simulink model "simple_eventbased"  (R2019a)
settings: Solver=VariableStepAuto  StartTime=0.0  StopTime=10.0  RelTol=1e-3  EnableMultiTasking=on
undefined symbols (not defined in the file or in its folder): genNext, m, n
settings Model: Creator=The MathWorks, Inc.  LastModifiedBy=The MathWorks, Inc.
settings DataIOCC: LimitDataPoints=on  ReturnWorkspaceOutputs=off
settings OptimizationCC: LifeSpan=inf
settings DebuggingCC: AllowSymbolicDim=off  SFUnexpectedBacktrackingDiag=warning  SFNoUnconditionalDefaultTransitionDiag=warning  SFExecutionAtInitializationDiag=none  ArithmeticOperatorsInVariantConditions=warning
settings ModelReferenceCC: PropagateSignalLabelsOutOfModel=off
settings SFSimCC: SimUseLocalCustomCode=off
settings RTWCC: RTWUseLocalCustomCode=off
settings CodeAppCC: StateflowObjectComments=on
settings GRTTargetCC: TargetLangStandard=C89/C90 (ANSI)
settings ConfigComp: CovMetricSettings=dw  CovHtmlReporting=on  CovSaveCumulativeToWorkspaceVar=on  CovSaveSingleToWorkspaceVar=on  CovExternalEMLEnable=off

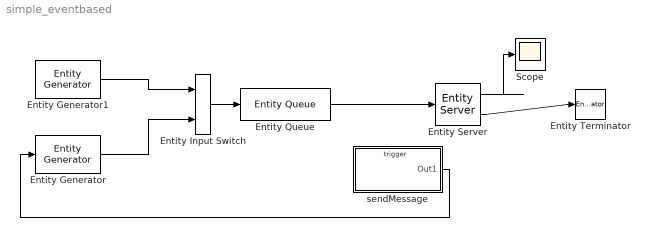
== system simple_eventbased ==
  Entity Input Switch : EntityInputSwitch  InputPortMessageModes=m,m  OutputPortMessageModes=m
  Entity Generator : EntityGenerator  InputPortMessageModes=m  OutputPortMessageModes=m  GenerationMethod=Event-based  EntityType=Structured  EntityTypeName=Entity
      settings: InputPortMap=u0
  Entity Generator1 : EntityGenerator  OutputPortMessageModes=m  Period=inf  EntityType=Structured  EntityTypeName=Entity
  Entity Queue : EntityQueue  InputPortMessageModes=m  OutputPortMessageModes=m
      settings: OutputPortMap=o5
  Entity Server : EntityServer  InputPortMessageModes=m  OutputPortMessageModes=n,m  Capacity=1  NumberEntitiesDeparted=on
      settings: OutputPortMap=o0,o9
  Entity Terminator : EntityTerminator  InputPortMessageModes=m  EntryAction=genNext();
  Scope : Scope
  sendMessage : Subsystem  TreatAsAtomicUnit=on
  wires:
  Entity Queue/1 -> Entity Server/1
  Entity Server/2 -> Entity Terminator/1
  Entity Input Switch/1 -> Entity Queue/1
  Entity Server/1 -> Scope/1
  sendMessage/1(Out1) -> Entity Generator/1
  Entity Generator/1 -> Entity Input Switch/2
  Entity Generator1/1 -> Entity Input Switch/1

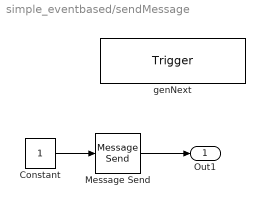
== system simple_eventbased/sendMessage ==
  genNext : TriggerPort  TriggerType=function-call  IsSimulinkFunction=on  FunctionName=genNext  VariantControl=Variant
  Constant : Constant
  Message Send : MessageSend  OutputPortMessageModes=m
      settings: InputPortMap=u1
  Out1 : Outport
  wires:
  Constant/1 -> Message Send/1
  Message Send/1 -> Out1/1
